simulink library "uavsimBlockset_alphabetaVa2uvw"  (Simulink 8.4)
settings: Solver=ode45  StartTime=0.0  StopTime=10.0  RelTol=1e-3
libraries: aerolibtransform2 x1
settings Model: Creator=mstolle  LastModifiedBy=j.bolting

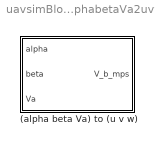
== system uavsimBlockset_alphabetaVa2uvw ==
  (alpha beta Va) to (u v w) : Subsystem

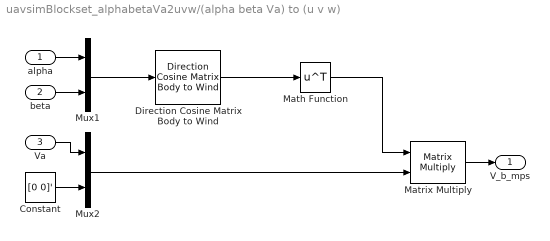
== system uavsimBlockset_alphabetaVa2uvw/(alpha beta Va) to (u v w) ==
  alpha : Inport
  beta : Inport  Port=2
  Va : Inport  Port=3
  Constant : Constant  Value=[0 0]'
  Direction Cosine Matrix Body to Wind : aerolibtransform2/Direction Cosine Matrix Body to Wind
  Math Function : Math  Operator=transpose  SaturateOnIntegerOverflow=on
  Matrix Multiply : Product  Multiplication=Matrix(*)
  Mux1 : Mux  Inputs=2
  Mux2 : Mux  Inputs=2
  V_b_mps : Outport
  wires:
  Matrix Multiply/1 -> V_b_mps/1
  alpha/1 -> Mux1/1
  beta/1 -> Mux1/2
  Mux1/1 -> Direction Cosine Matrix Body to Wind/1
  Va/1 -> Mux2/1
  Constant/1 -> Mux2/2
  Direction Cosine Matrix Body to Wind/1 -> Math Function/1
  Mux2/1 -> Matrix Multiply/2
  Math Function/1 -> Matrix Multiply/1
